simulink model "DinamicaInversa"  (R2014b)
settings: Solver=ode45  StartTime=0.0  StopTime=Tf+0.001  RelTol=1e-3
InitFcn:
  | clear all
  | InizializzazioneDinamicaInversa
StopFcn:
  | plot(errVel)
  | title('Errore in velocità')
  | legend('joint1','joint2','joint3','joint4','joint5','joint6')
  | grid
  | figure
  | plot(errPos)
  | title('Errore in Posizione')
  | legend('joint1','joint2','joint3','joint4','joint5','joint6')
  | grid
undefined symbols (not defined in the file): invRa, Kd, Kp, kr, Kt, kv, q0, qp0, T
settings Model: Creator=Sabatino  LastModifiedBy=Sabatino

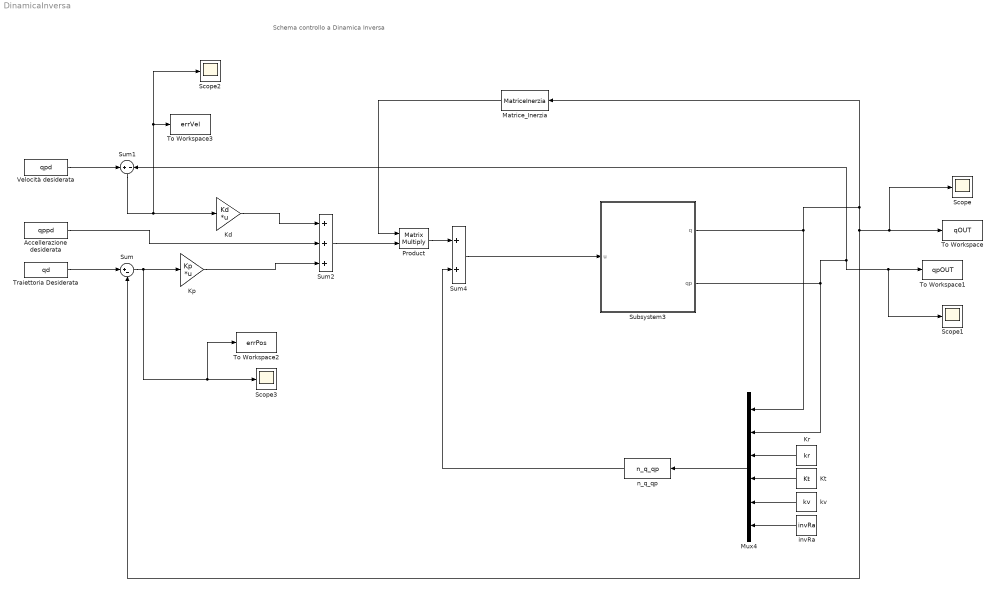
== system DinamicaInversa ==
  note: Schema controllo a Dinamica Inversa
  Accellerazione desiderata : FromWorkspace  VariableName=qppd  SampleTime=T
  Kd : Gain  Gain=Kd  Multiplication=Matrix(K*u)
  Kp : Gain  Gain=Kp  Multiplication=Matrix(K*u)
  Kr : Constant  Value=kr
  Kt : Constant  Value=Kt
  Matrice_Inerzia : MATLABFcn  MATLABFcn=MatriceInerzia  Output1D=off
  Mux4 : Mux  Inputs=6
  Product : Product  Multiplication=Matrix(*)
  Scope{,1..3} (4 alike) : Scope
      Scope settings: YMin=-2.5  YMax=2
      Scope1 settings: YMin=-8  YMax=4
      Scope2 settings: YMin=-0.00035  YMax=0.00015  SaveName=ScopeData2
      Scope3 settings: YMin=-0.0006  YMax=0.0006  SaveName=ScopeData3
  Subsystem3 : Subsystem
      mask Display:
      | disp('Manipolatore');
      | port_label('input', 1, 'u');
      | port_label('output', 1, 'q');
      | port_label('output', 2, 'qp');
  Sum : Sum  Inputs=|+-
  Sum1 : Sum  Inputs=+|-
  Sum2 : Sum  Inputs=+++
  Sum4 : Sum
  To Workspace : ToWorkspace  VariableName=qOUT  SaveFormat=Timeseries  SampleTime=-1
  To Workspace1 : ToWorkspace  VariableName=qpOUT  SaveFormat=Timeseries  SampleTime=-1
  To Workspace2 : ToWorkspace  VariableName=errPos  SaveFormat=Timeseries  SampleTime=-1
  To Workspace3 : ToWorkspace  VariableName=errVel  SaveFormat=Timeseries  SampleTime=-1
  Traiettoria Desiderata : FromWorkspace  VariableName=qd  SampleTime=T
  Velocità desiderata : FromWorkspace  VariableName=qpd  SampleTime=T
  invRa : Constant  Value=invRa
  kv : Constant  Value=kv
  n_q_qp : MATLABFcn  MATLABFcn=n_q_qp  OutputDimensions=6
  wires:
  Traiettoria Desiderata/1 -> Sum/1
  Sum/1 -> To Workspace2/1, Scope3/1, Kp/1
  Subsystem3/1(q) -> Mux4/1, Sum/2, Scope/1, To Workspace/1, Matrice_Inerzia/1
  Subsystem3/2(qp) -> Mux4/2, Sum1/2, To Workspace1/1, Scope1/1
  Kp/1 -> Sum2/3
  Velocità desiderata/1 -> Sum1/1
  Sum1/1 -> To Workspace3/1, Scope2/1, Kd/1
  Kd/1 -> Sum2/1
  Accellerazione desiderata/1 -> Sum2/2
  Sum2/1 -> Product/2
  Matrice_Inerzia/1 -> Product/1
  Product/1 -> Sum4/1
  n_q_qp/1 -> Sum4/2
  Sum4/1 -> Subsystem3/1(u)
  Mux4/1 -> n_q_qp/1
  Kr/1 -> Mux4/3
  Kt/1 -> Mux4/4
  kv/1 -> Mux4/5
  invRa/1 -> Mux4/6

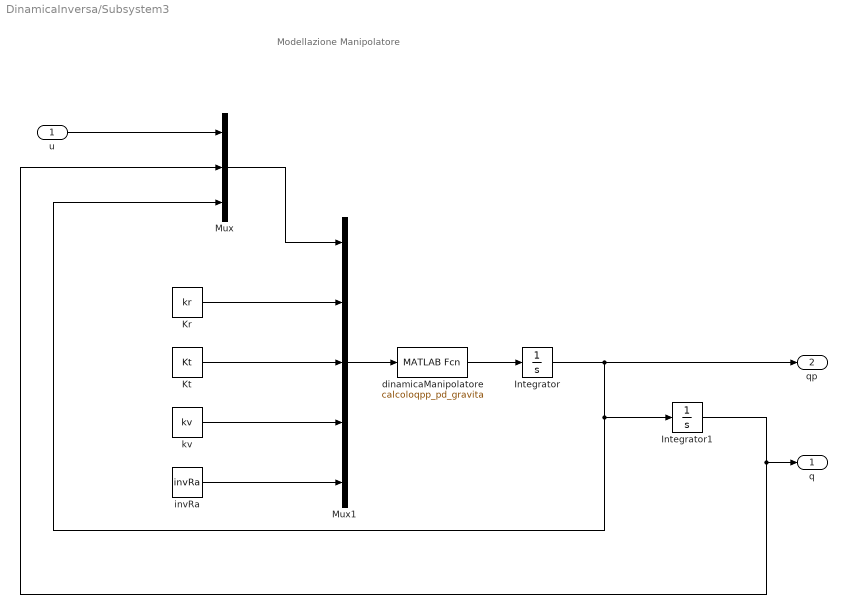
== system DinamicaInversa/Subsystem3 ==
  note: Modellazione Manipolatore
  u : Inport
  Integrator : Integrator  InitialCondition=qp0
  Integrator1 : Integrator  InitialCondition=q0
  Kr : Constant  Value=kr
  Kt : Constant  Value=Kt
  Mux : Mux  Inputs=3
  Mux1 : Mux  Inputs=5
  dinamicaManipolatore : MATLABFcn  MATLABFcn=calcoloqpp_pd_gravita  OutputDimensions=6
  invRa : Constant  Value=invRa
  kv : Constant  Value=kv
  q : Outport
  qp : Outport  Port=2
  wires:
  u/1 -> Mux/1
  Mux/1 -> Mux1/1
  dinamicaManipolatore/1 -> Integrator/1
  Integrator/1 -> Mux/3, Integrator1/1, qp/1
  Integrator1/1 -> Mux/2, q/1
  Kr/1 -> Mux1/2
  Kt/1 -> Mux1/3
  kv/1 -> Mux1/4
  invRa/1 -> Mux1/5
  Mux1/1 -> dinamicaManipolatore/1
